simulink model "mpc555rt_iohost"  (Simulink 6.0)
settings: Solver=FixedStepDiscrete  StartTime=0.0  StopTime=inf  RelTol=1e-3
libraries: vector_candrivers x9, canblocks x8, mpc555extras x1
settings Model: Creator=The MathWorks Inc.  LastModifiedBy=batserve  ExtModeAutoUpdateStatusClock=off  ProdHWDeviceType=Specified
settings DataIOCC: SignalLoggingName=sigsOut
settings OptimizationCC: BooleanDataType=off  InlineInvariantSignals=off
settings DebuggingCC: CheckExecutionContextPreStartOutputMsg=on  CheckExecutionContextRuntimeOutputMsg=on  SolverPrmCheckMsg=none
settings HardwareCC: ProdHWDeviceType=Specified

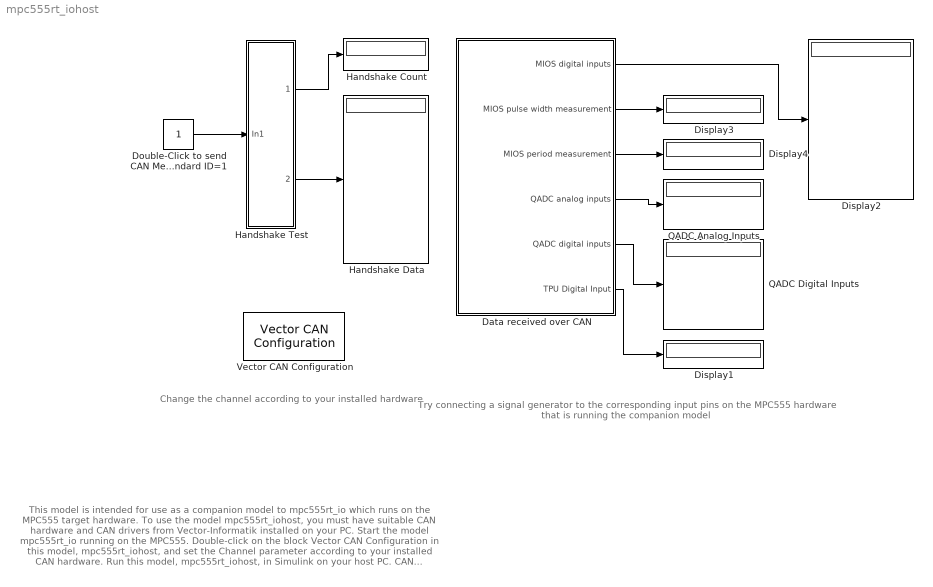
== system mpc555rt_iohost ==
  note: This model is intended for use as a companion model to mpc555rt_io which runs on the MPC555
      | target hardware. To use the model mpc555rt_iohost, you must have suitable CAN hardware and
      | CAN drivers from Vector-Informatik installed on your PC.
      |
      | Start the model mpc555rt_io running on the MPC555.
      |
      | Double-click on the block Vector CAN Configuration in this model, mpc555rt_iohost,  and set the
      | Channel parameter according to your installed CAN hardware.
      |
      | Run this model, mpc555rt_iohost, in Simulink on your host PC.
      |
      | CAN messages are received from the MPC555 and displayed in the numeric display blocks above.
  note: Change the channel according
      | to your installed hardware
  note: Try connecting a signal generator to the
      | corresponding input pins on the MPC555 hardware
      | that is running the companion model
  " Vector CAN Configuration  " : vector_candrivers/ Vector CAN Configuration  tag_param=config1  channel_param=None
  Data received over CAN : Subsystem  PropExecContextAcrossSSBoundary=on
  Display{1..4} (4 alike) : Display
  Double-Click to send CAN Message with Standard ID=1 : Constant
      settings: OpenFcn=if strcmp(get_param(gcb,'value'),'1'), set_param(gcb,'value','-1'); else set_param(gcb,'value','1'); end
  Handshake Count : Display
  Handshake Data : Display
  Handshake Test : Subsystem  PropExecContextAcrossSSBoundary=on
  QADC Analog Inputs : Display
  QADC Digital Inputs : Display
  wires:
  Double-Click to send CAN Message with Standard ID=1/1 -> Handshake Test/1(In1)
  Data received over CAN/4(QADC analog inputs) -> QADC Analog Inputs/1
  Data received over CAN/5(QADC digital inputs) -> QADC Digital Inputs/1
  Data received over CAN/1(MIOS digital inputs) -> Display2/1
  Data received over CAN/2(MIOS pulse width measurement) -> Display3/1
  Handshake Test/1(count) -> Handshake Count/1
  Handshake Test/2(data) -> Handshake Data/1
  Data received over CAN/3("MIOS period measurement ") -> Display4/1
  Data received over CAN/6(TPU Digital Input) -> Display1/1

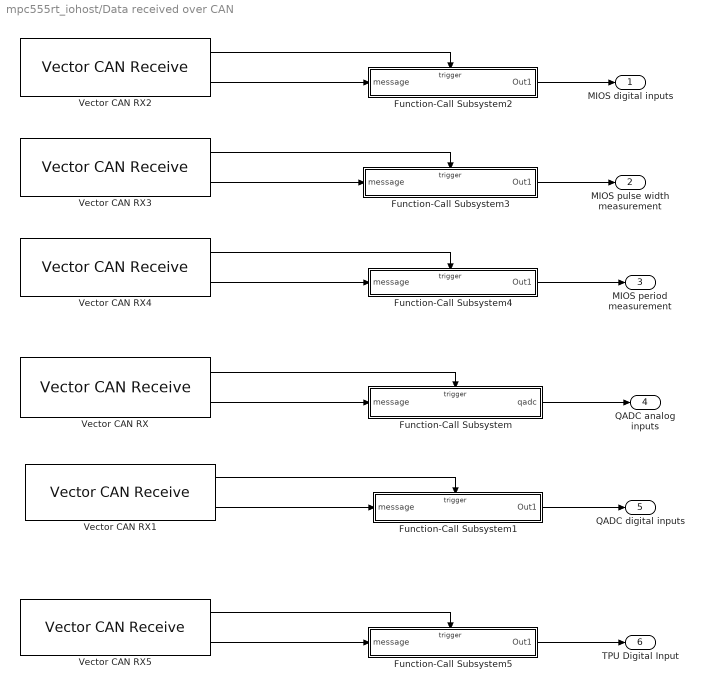
== system mpc555rt_iohost/Data received over CAN ==
  Function-Call Subsystem : Subsystem  TreatAsAtomicUnit=on  PropExecContextAcrossSSBoundary=on
  Function-Call Subsystem1 : Subsystem  TreatAsAtomicUnit=on  PropExecContextAcrossSSBoundary=on
  Function-Call Subsystem2 : Subsystem  TreatAsAtomicUnit=on  PropExecContextAcrossSSBoundary=on
  Function-Call Subsystem3 : Subsystem  TreatAsAtomicUnit=on  PropExecContextAcrossSSBoundary=on
  Function-Call Subsystem4 : Subsystem  TreatAsAtomicUnit=on  PropExecContextAcrossSSBoundary=on
  Function-Call Subsystem5 : Subsystem  TreatAsAtomicUnit=on  PropExecContextAcrossSSBoundary=on
  Vector CAN RX : vector_candrivers/Vector CAN Receive  Tag=config1  tag_param=config1  ids=3  frame_type_in=Extended (29-bit identifier)  sample_time=1  output_time=off  loop=off
  Vector CAN RX1 : vector_candrivers/Vector CAN Receive  Tag=config1  tag_param=config1  ids=[5]  frame_type_in=Extended (29-bit identifier)  sample_time=1  output_time=off  loop=off
  Vector CAN RX2 : vector_candrivers/Vector CAN Receive  Tag=config1  tag_param=config1  ids=4  frame_type_in=Extended (29-bit identifier)  sample_time=1  output_time=off  loop=off
  Vector CAN RX3 : vector_candrivers/Vector CAN Receive  Tag=config1  tag_param=config1  ids=1  frame_type_in=Extended (29-bit identifier)  sample_time=1  output_time=off  loop=off
  Vector CAN RX4 : vector_candrivers/Vector CAN Receive  Tag=config1  tag_param=config1  ids=2  frame_type_in=Extended (29-bit identifier)  sample_time=1  output_time=off  loop=off
  Vector CAN RX5 : vector_candrivers/Vector CAN Receive  Tag=config1  tag_param=config1  ids=[6]  frame_type_in=Extended (29-bit identifier)  sample_time=1  output_time=off  loop=off
  MIOS digital inputs : Outport
  MIOS pulse width measurement : Outport  Port=2
  "MIOS period measurement " : Outport  Port=3
  QADC analog inputs : Outport  Port=4
  QADC digital inputs : Outport  Port=5
  TPU Digital Input : Outport  Port=6
  wires:
  Vector CAN RX2/2 -> Function-Call Subsystem2/1(message)
  Vector CAN RX2/1 -> Function-Call Subsystem2/Trigger
  Function-Call Subsystem3/1(Out1) -> MIOS pulse width measurement/1
  Function-Call Subsystem4/1(Out1) -> "MIOS period measurement "/1
  Vector CAN RX/1 -> Function-Call Subsystem/Trigger
  Vector CAN RX/2 -> Function-Call Subsystem/1(message)
  Vector CAN RX1/1 -> Function-Call Subsystem1/Trigger
  Vector CAN RX1/2 -> Function-Call Subsystem1/1(message)
  Function-Call Subsystem/1(qadc) -> QADC analog inputs/1
  Function-Call Subsystem1/1(Out1) -> QADC digital inputs/1
  Function-Call Subsystem2/1(Out1) -> MIOS digital inputs/1
  Vector CAN RX3/2 -> Function-Call Subsystem3/1(message)
  Vector CAN RX3/1 -> Function-Call Subsystem3/Trigger
  Vector CAN RX4/2 -> Function-Call Subsystem4/1(message)
  Vector CAN RX4/1 -> Function-Call Subsystem4/Trigger
  Vector CAN RX5/2 -> Function-Call Subsystem5/1(message)
  Vector CAN RX5/1 -> Function-Call Subsystem5/Trigger
  Function-Call Subsystem5/1(Out1) -> TPU Digital Input/1

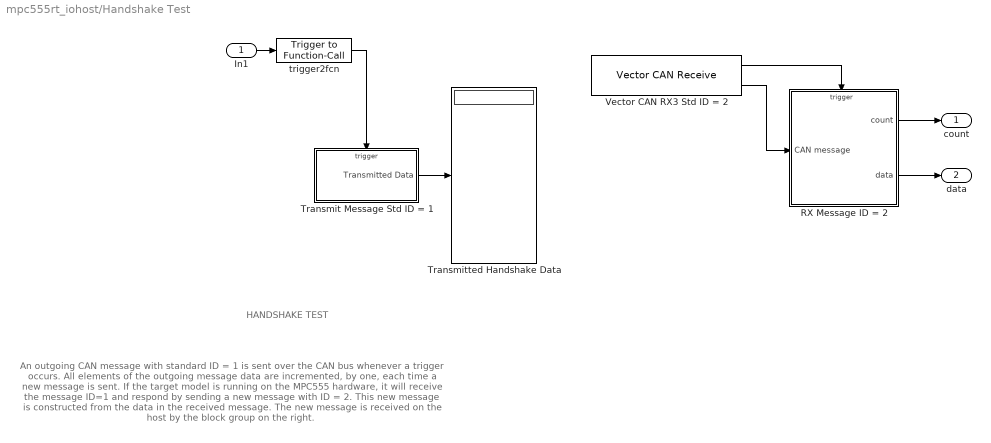
== system mpc555rt_iohost/Handshake Test ==
  note: HANDSHAKE TEST
  note: An outgoing CAN message with standard ID = 1 is sent over the CAN bus whenever a trigger occurs.  All elements of the outgoing message data
      | are incremented, by one, each time a new message is sent.
      |
      | If the target model is running on the MPC555 hardware, it will receive the message ID=1 and respond by sending a new message with ID = 2.
      | This new message is constructed from the data in the received message.
      |
      | The new message is received on the host by the block group on the right.
  In1 : Inport  Port=1  LatchInput=off
  RX Message ID = 2 : Subsystem  TreatAsAtomicUnit=on  PropExecContextAcrossSSBoundary=on
  Transmit Message Std ID = 1 : Subsystem  TreatAsAtomicUnit=on  PropExecContextAcrossSSBoundary=on
  Transmitted Handshake Data : Display
  Vector CAN RX3 Std ID = 2 : vector_candrivers/Vector CAN Receive  Tag=config1  tag_param=config1  ids=[2]  frame_type_in=Standard (11-bit identifier)  sample_time=1  output_time=off  loop=off
  trigger2fcn : mpc555extras/Trigger to Function-Call
  count : Outport
  data : Outport  Port=2
  wires:
  trigger2fcn/1 -> Transmit Message Std ID = 1/Trigger
  Vector CAN RX3 Std ID = 2/1 -> RX Message ID = 2/Trigger
  Vector CAN RX3 Std ID = 2/2 -> RX Message ID = 2/1(CAN message)
  In1/1 -> trigger2fcn/1
  RX Message ID = 2/1(count) -> count/1
  RX Message ID = 2/2(data) -> data/1
  Transmit Message Std ID = 1/1(Transmitted Data) -> Transmitted Handshake Data/1

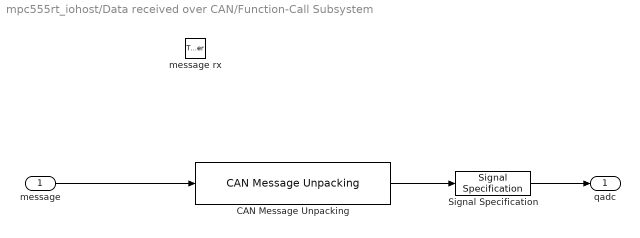
== system mpc555rt_iohost/Data received over CAN/Function-Call Subsystem ==
  message : Inport  Port=1  LatchInput=off
  message rx : TriggerPort  TriggerType=function-call  ZeroCross=off
  CAN Message Unpacking : canblocks/CAN Message Unpacking/CAN Message Unpacking  showData=on  showID=off  showLength=off  endian=Big Endian (Motorola)
  Signal Specification : SignalSpecification  Dimensions=2  DataType=single
  qadc : Outport
  wires:
  message/1 -> CAN Message Unpacking/1
  CAN Message Unpacking/1 -> Signal Specification/1
  Signal Specification/1 -> qadc/1

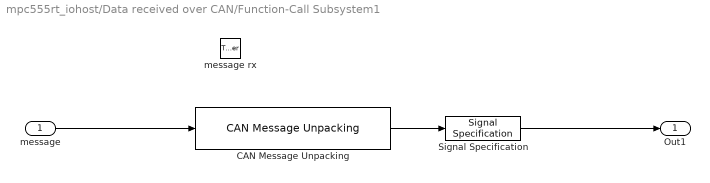
== system mpc555rt_iohost/Data received over CAN/Function-Call Subsystem1 ==
  message : Inport  Port=1  LatchInput=off
  message rx : TriggerPort  TriggerType=function-call  ZeroCross=off
  CAN Message Unpacking : canblocks/CAN Message Unpacking/CAN Message Unpacking  showData=on  showID=off  showLength=off  endian=Big Endian (Motorola)
  Signal Specification : SignalSpecification  Dimensions=4  DataType=uint8
  Out1 : Outport
  wires:
  message/1 -> CAN Message Unpacking/1
  CAN Message Unpacking/1 -> Signal Specification/1
  Signal Specification/1 -> Out1/1

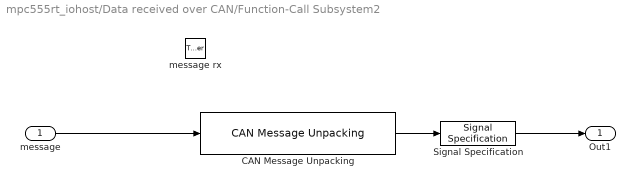
== system mpc555rt_iohost/Data received over CAN/Function-Call Subsystem2 ==
  message : Inport  Port=1  LatchInput=off
  message rx : TriggerPort  TriggerType=function-call  ZeroCross=off
  CAN Message Unpacking : canblocks/CAN Message Unpacking/CAN Message Unpacking  showData=on  showID=off  showLength=off  endian=Big Endian (Motorola)
  Signal Specification : SignalSpecification  Dimensions=8  DataType=uint8
  Out1 : Outport
  wires:
  message/1 -> CAN Message Unpacking/1
  CAN Message Unpacking/1 -> Signal Specification/1
  Signal Specification/1 -> Out1/1

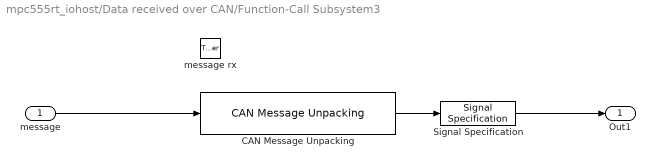
== system mpc555rt_iohost/Data received over CAN/Function-Call Subsystem3 ==
  message : Inport  Port=1  LatchInput=off
  message rx : TriggerPort  TriggerType=function-call  ZeroCross=off
  CAN Message Unpacking : canblocks/CAN Message Unpacking/CAN Message Unpacking  showData=on  showID=off  showLength=off  endian=Big Endian (Motorola)
  Signal Specification : SignalSpecification  Dimensions=1  DataType=single
  Out1 : Outport
  wires:
  message/1 -> CAN Message Unpacking/1
  CAN Message Unpacking/1 -> Signal Specification/1
  Signal Specification/1 -> Out1/1

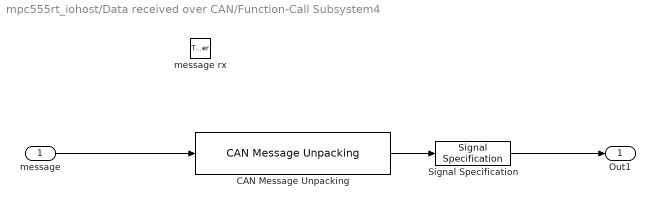
== system mpc555rt_iohost/Data received over CAN/Function-Call Subsystem4 ==
  message : Inport  Port=1  LatchInput=off
  message rx : TriggerPort  TriggerType=function-call  ZeroCross=off
  CAN Message Unpacking : canblocks/CAN Message Unpacking/CAN Message Unpacking  showData=on  showID=off  showLength=off  endian=Big Endian (Motorola)
  Signal Specification : SignalSpecification  Dimensions=1  DataType=single
  Out1 : Outport
  wires:
  message/1 -> CAN Message Unpacking/1
  CAN Message Unpacking/1 -> Signal Specification/1
  Signal Specification/1 -> Out1/1

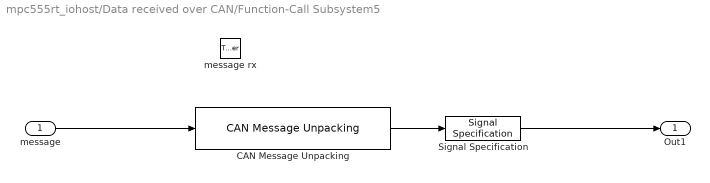
== system mpc555rt_iohost/Data received over CAN/Function-Call Subsystem5 ==
  message : Inport  Port=1  LatchInput=off
  message rx : TriggerPort  TriggerType=function-call  ZeroCross=off
  CAN Message Unpacking : canblocks/CAN Message Unpacking/CAN Message Unpacking  showData=on  showID=off  showLength=off  endian=Big Endian (Motorola)
  Signal Specification : SignalSpecification  Dimensions=1  DataType=uint8
  Out1 : Outport
  wires:
  Signal Specification/1 -> Out1/1
  CAN Message Unpacking/1 -> Signal Specification/1
  message/1 -> CAN Message Unpacking/1

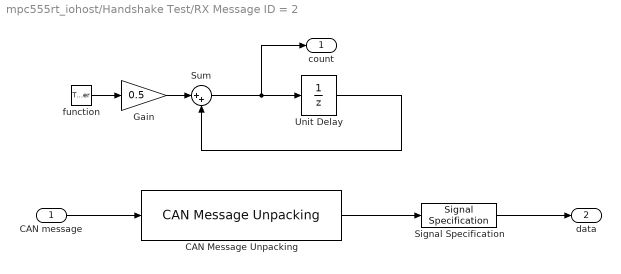
== system mpc555rt_iohost/Handshake Test/RX Message ID = 2 ==
  CAN message : Inport  Port=1  LatchInput=off
  function : TriggerPort  TriggerType=function-call  ShowOutputPort=on  ZeroCross=off
  CAN Message Unpacking : canblocks/CAN Message Unpacking/CAN Message Unpacking  showData=on  showID=off  showLength=off  endian=Big Endian (Motorola)
  Gain : Gain  Gain=0.5  SaturateOnIntegerOverflow=on
  Signal Specification : SignalSpecification  Dimensions=8  DataType=uint8
  Sum : Sum  Inputs=|++  SaturateOnIntegerOverflow=on  InputSameDT=on
  Unit Delay : UnitDelay  SampleTime=-1
  count : Outport
  data : Outport  Port=2
  wires:
  function/1 -> Gain/1
  Sum/1 -> Unit Delay/1, count/1
  Unit Delay/1 -> Sum/2
  CAN message/1 -> CAN Message Unpacking/1
  CAN Message Unpacking/1 -> Signal Specification/1
  Signal Specification/1 -> data/1
  Gain/1 -> Sum/1

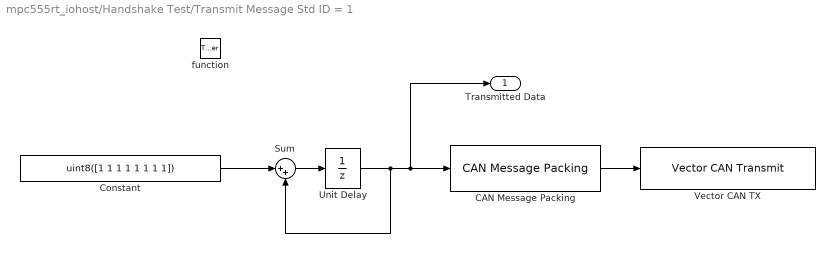
== system mpc555rt_iohost/Handshake Test/Transmit Message Std ID = 1 ==
  function : TriggerPort  TriggerType=function-call  ZeroCross=off
  CAN Message Packing : canblocks/CAN Message Packing  id=1  message_type=Standard (11-bit identifier)  endian=Big Endian (Motorola)
  Constant : Constant  Value=uint8([1 1 1 1 1 1 1 1])
  Sum : Sum  Inputs=|++  SaturateOnIntegerOverflow=on  InputSameDT=on
  Unit Delay : UnitDelay  X0=uint8([1 2 3 4 5 6 7 8])  SampleTime=-1
  Vector CAN TX : vector_candrivers/Vector CAN Transmit  Tag=config1  tag_param=config1  sample_time=-1
  Transmitted Data : Outport  InitialOutput=uint8([1 2 3 4 5 6 7 8])
  wires:
  CAN Message Packing/1 -> Vector CAN TX/1
  Sum/1 -> Unit Delay/1
  Unit Delay/1 -> Sum/2, Transmitted Data/1, CAN Message Packing/1
  Constant/1 -> Sum/1
